simulink model "P3k1"  (R2017b)
settings: Solver=VariableStepAuto  StartTime=0.0  StopTime=10.0  RelTol=1e-3
values from neighbouring files (symbols this model uses):
  a = [ -0.0000 1.0000 -0.0000 -0.0000 ... (first row only)    [P3a.m]
  b = [ -0.0000 0.0000 ... (first row only)    [P3a.m]
  c = [ 1.0000 -0.0050 0.0000 0.0000 ... (first row only)    [P3a.m]
  P0 = 1000 * eye(4)    [P3a.m]
undefined symbols (not defined in the file or in its folder): K, l
settings Model: Creator=Soutrik  LastModifiedBy=Soutrik

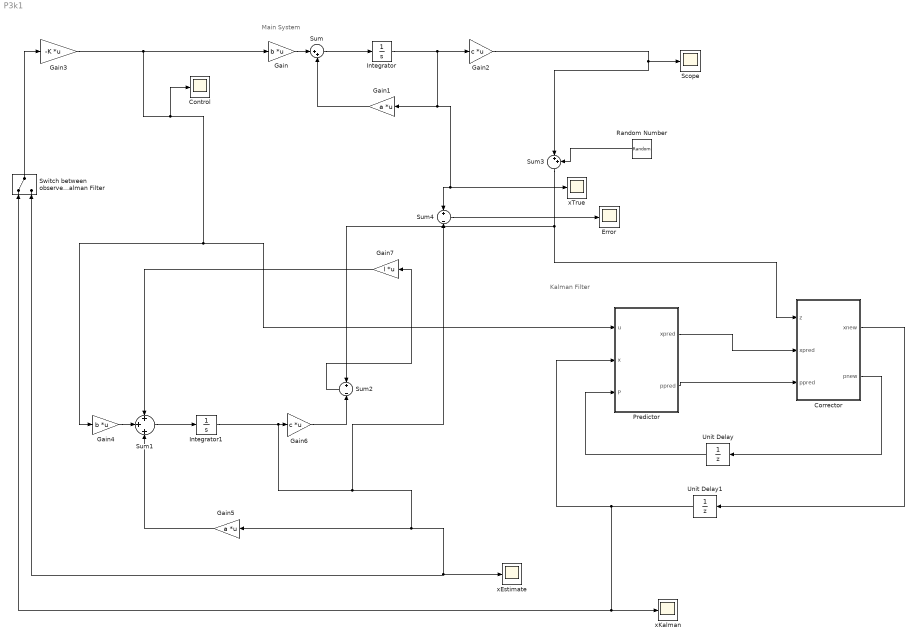
== system P3k1 ==
  note: Kalman Filter
  note: Main System
  Control : Scope
  Corrector : MATLAB Function  TreatAsAtomicUnit=on
  Error : Scope
  Gain : Gain  Gain=b  Multiplication=Matrix(K*u)
  Gain1 : Gain  Gain=a  Multiplication=Matrix(K*u)
  Gain2 : Gain  Gain=c  Multiplication=Matrix(K*u)
  Gain3 : Gain  Gain=-K  Multiplication=Matrix(K*u)
  Gain4 : Gain  Gain=b  Multiplication=Matrix(K*u)
  Gain5 : Gain  Gain=a  Multiplication=Matrix(K*u)
  Gain6 : Gain  Gain=c  Multiplication=Matrix(K*u)
  Gain7 : Gain  Gain=l  Multiplication=Matrix(K*u)
  Integrator : Integrator  InitialCondition=[0.02 0 0 0]
  Integrator1 : Integrator  InitialCondition=[0.02 0 0 0]
  Predictor : MATLAB Function  TreatAsAtomicUnit=on
  Random Number : RandomNumber  Variance=[0.000001, 0.000001, 0.000001, 0.000001]  Seed=[1 2 3 4]  SampleTime=0.01
  Scope : Scope
  Sum : Sum  Inputs=|++
  Sum1 : Sum  Inputs=+|+|+
  Sum2 : Sum  Inputs=+||-
  Sum3 : Sum  Inputs=|++
  Sum4 : Sum  Inputs=+||-
  Switch between observer and Kalman Filter : ManualSwitch
  Unit Delay : UnitDelay  InitialCondition=P0  SampleTime=-1
  Unit Delay1 : UnitDelay  InitialCondition=[0 0 0 0]  SampleTime=-1
  xEstimate : Scope
  xKalman : Scope
  xTrue : Scope
  wires:
  Sum4/1 -> Error/1
  Sum2/1 -> Gain7/1
  Gain7/1 -> Sum1/1
  Gain6/1 -> Sum2/2
  Switch between observer and Kalman Filter/1 -> Gain3/1
  Integrator1/1 -> Sum4/2, Switch between observer and Kalman Filter/2, xEstimate/1, Gain5/1, Gain6/1
  Sum1/1 -> Integrator1/1
  Gain5/1 -> Sum1/3
  Gain4/1 -> Sum1/2
  Random Number/1 -> Sum3/2
  Unit Delay1/1 -> Predictor/2(x), xKalman/1, Switch between observer and Kalman Filter/1
  Integrator/1 -> xTrue/1, Sum4/1, Gain1/1, Gain2/1
  Gain2/1 -> Sum3/1, Scope/1
  Sum/1 -> Integrator/1
  Gain1/1 -> Sum/2
  Gain/1 -> Sum/1
  Predictor/2(ppred) -> Corrector/3(ppred)
  Corrector/1(xnew) -> Unit Delay1/1
  Corrector/2(pnew) -> Unit Delay/1
  Unit Delay/1 -> Predictor/3(P)
  Predictor/1(xpred) -> Corrector/2(xpred)
  Sum3/1 -> Corrector/1(z), Sum2/1
  Gain3/1 -> Predictor/1(u), Gain4/1, Control/1, Gain/1

== matlab function P3k1/Corrector ==
  data: z input size=4; xpred input size=[4 1]; xnew output size=4; ppred input size=[4 4]; pnew output size=[4 4]
%% Corrector algorithm
function [xnew,pnew]= corrector(z, xpred, ppred)
R=0.0001*eye(4);
%R = eye(4);
C = [ 1.0000 -0.0050 0.0000 0.0000;
    0.0000 1.0025 0.0000 -0.0000;
    0.1604 0.0084 0.9612 0.2769;
    0.0000 -0.0049 -0.0011 0.0040 ];
H=C;
k=ppred*H'*inv((H*ppred*H')+R);
pnew=((eye(4)-k*H)*ppred*transpose(eye(4)-k*H))+k*R*k';
xnew=xpred+k*(z-H*xpred);
end

== matlab function P3k1/Predictor ==
  data: u input size=2; xpred output size=4; x input size=4; ppred output size=[4 4]; P input size=[4 4]
%% Predictor algorithm
function [xpred, ppred]= predictor(u,x,P)
a = [0 1;-1 -0.7];
b = [0;1];
Q=10*eye(2);
R=eye(2);

ad=expm(a*0.01);
bd=inv(a)*(ad-eye(4))*b;

F=[-a Q;zeros(2) a'];
G=expm(F*0.01);
Glr=G(3:4,3:4);
Gur=G(1:2,3:4);
Qd=Glr'*Gur;

xpred=ad*x+bd*u;
ppred=ad*P+ad'*Qd;
end
